simulink model "BD_PAR_SimplorerDemo"  (Simulink 4.1.1)
settings: Solver=ode1  SolverMode=SingleTasking  StartTime=0.0  StopTime=max(cyc_mph(:,1))  FixedStep=1  MaxStep=1  RelTol=1e-3  AbsTol=1e-3
undefined symbols (not defined in the file): ex_calc, fc_emis, fc_max_trq, fc_trq_scale
libraries: lib_transmission x4, lib_wheel x2, lib_controls x2, lib_help x2, lib_outputs x1, lib_interactive x1, lib_drive_cycle x1, lib_energy_storage x1, lib_exhaust x1, lib_fuel_converter x1, lib_electric_machine x1, lib_power_bus x1
settings Model: LastModifiedBy=ssprik  SaveTime=off  SaveOutput=off  LimitDataPoints=off  UnconnectedLineMsg=none  RTWTemplateMakefile=grt_vc.tmf  ExtModeTrigMode=oneshot  ExtModeArmWhenConnect=off

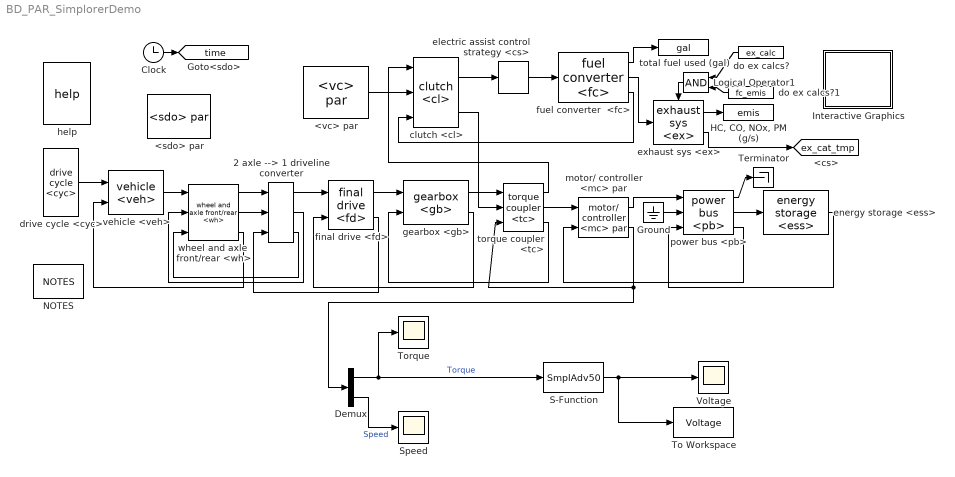
== system BD_PAR_SimplorerDemo ==
  2 axle --> 1 driveline converter : lib_wheel/2 axle --> 1 driveline converter
      settings: RTWFcnNameOpts=Auto  RTWFileNameOpts=Auto
  <sdo> par : lib_outputs/<sdo> par
  <vc> par : lib_controls/<vc> par
      link override config traction control: BlockChoice=traction control
  Clock : Clock
      settings: DisplayTime=off  Decimation=10
  Demux : Demux  Outputs=2  BusSelectionMode=off
  Ground : Ground
  "HC, CO, NOx, PM (g/s)" : ToWorkspace  VariableName=emis  SampleTime=0  SaveFormat=Array
  Interactive Graphics : Subsystem  BlockChoice=off
      settings: AttributesFormatString=%<BlockChoice>  TemplateBlock=lib_interactive/Interactive Graphics  MemberBlocks=off,on  RTWFcnNameOpts=Auto  RTWFileNameOpts=Auto
  Logical Operator1 : Logic  Orientation=left  Operator=AND  Inputs=2
  NOTES : lib_help/NOTES
  S-Function : S-Function  FunctionName=SmplAdv50  Parameters=0,1.0  PortCounts=[]  SFunctionModules=''
  Speed : Scope
      settings: TimeRange=auto  YMin=0  YMax=550  SaveToWorkspace=off  SaveName=ScopeData2  LimitDataPoints=on  MaxDataPoints=5000
  Terminator : Terminator
  To Workspace : ToWorkspace  VariableName=Voltage  SampleTime=-1  SaveFormat=Array
  Torque : Scope
      settings: TimeRange=auto  YMin=-65  YMax=20  SaveToWorkspace=off  LimitDataPoints=on  MaxDataPoints=5000
  Voltage : Scope
      settings: TimeRange=1400  YMin=-5000  YMax=1000  SaveToWorkspace=off  SaveName=ScopeData  LimitDataPoints=on  MaxDataPoints=5000
  clutch <cl> : lib_transmission/clutch <cl>  slip_spd=vc_launch_spd  maxtrq=max(fc_max_trq)*fc_trq_scale
  do ex calcs? : Constant  Orientation=left  Value=ex_calc
  do ex calcs?1 : Constant  Orientation=left  Value=fc_emis
  drive cycle <cyc> : lib_drive_cycle/drive cycle <cyc>
  electric assist control strategy <cs> : lib_controls/electric assist control strategy <cs>
  energy storage <ess> : lib_energy_storage/energy storage <ess>  AncestorBlock=lib_energy_storage/Subsystem/energy storage <ess>
      link override ess config: BlockChoice=energy storage <ess>
  exhaust sys <ex> : lib_exhaust/exhaust sys <ex>
  final drive <fd> : lib_transmission/final drive <fd>
  fuel converter  <fc> : lib_fuel_converter/fuel converter  <fc>
      link override fuel use and EO emis Configurable Subsystem: BlockChoice=fuel use and EO emis
  gearbox <gb> : lib_transmission/gearbox <gb>
  help : lib_help/help
  motor/ controller <mc> par : lib_electric_machine/motor// controller <mc> par
  power bus <pb> : lib_power_bus/power bus <pb>
  torque coupler <tc> : lib_transmission/torque coupler <tc>
  total fuel used (gal) : ToWorkspace  VariableName=gal  SampleTime=0  SaveFormat=Array
  vehicle <veh> : lib_vehicle/vehicle <veh>
      link override rolling resistance force: BlockChoice=force req'd to overcome rolling resistance (N)
      link override vehicle speed: BlockChoice=vehicle speed (m/s)
  wheel and axle  front/rear <wh> : lib_wheel/wheel and axle  front//rear <wh>
  tag scope: ex_cat_tmp=global, time=global
  wires:
  final drive <fd>/1 -> gearbox <gb>/1
  drive cycle <cyc>/1 -> vehicle <veh>/1
  clutch <cl>/1 -> electric assist control strategy <cs>/1
  electric assist control strategy <cs>/1 -> fuel converter  <fc>/1
  fuel converter  <fc>/2 -> exhaust sys <ex>/1
  do ex calcs?/1 -> Logical Operator1/1
  fuel converter  <fc>/3 -> clutch <cl>/3
  fuel converter  <fc>/1 -> total fuel used (gal)/1
  exhaust sys <ex>/1 -> "HC, CO, NOx, PM (g/s)"/1
  Logical Operator1/1 -> exhaust sys <ex>/Enable
  do ex calcs?1/1 -> Logical Operator1/2
  Clock/1 -> [time]
  gearbox <gb>/2 -> final drive <fd>/2
  torque coupler <tc>/3 -> gearbox <gb>/2
  torque coupler <tc>/1 -> clutch <cl>/1
  clutch <cl>/2 -> torque coupler <tc>/2
  gearbox <gb>/1 -> torque coupler <tc>/1
  <vc> par/1 -> clutch <cl>/2
  motor/ controller <mc> par/2 -> torque coupler <tc>/3, Demux/1
  motor/ controller <mc> par/1 -> power bus <pb>/1
  Ground/1 -> power bus <pb>/2
  power bus <pb>/3 -> motor/ controller <mc> par/2
  power bus <pb>/2 -> energy storage <ess>/1
  power bus <pb>/1 -> Terminator/1
  energy storage <ess>/1 -> power bus <pb>/3
  torque coupler <tc>/2 -> motor/ controller <mc> par/1
  exhaust sys <ex>/2 -> [ex_cat_tmp]
  Demux/1 -> S-Function/1, Torque/1  "Torque"
  Demux/2 -> Speed/1  "Speed"
  S-Function/1 -> Voltage/1, To Workspace/1
  vehicle <veh>/1 -> wheel and axle  front/rear <wh>/1
  wheel and axle  front/rear <wh>/1 -> 2 axle --> 1 driveline converter/1
  wheel and axle  front/rear <wh>/2 -> 2 axle --> 1 driveline converter/2
  2 axle --> 1 driveline converter/1 -> final drive <fd>/1
  2 axle --> 1 driveline converter/2 -> wheel and axle  front/rear <wh>/2
  2 axle --> 1 driveline converter/3 -> wheel and axle  front/rear <wh>/3
  final drive <fd>/2 -> 2 axle --> 1 driveline converter/3
  wheel and axle  front/rear <wh>/3 -> vehicle <veh>/2

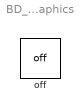
== system BD_PAR_SimplorerDemo/Interactive Graphics ==
  off : lib_interactive/off  Tag=Altia_off  Orientation=up
